simulink model "Zhongxiang_control"  (R2016a)
settings: Solver=VariableStepAuto  StartTime=0.0  StopTime=60  RelTol=1e-3
undefined symbols (not defined in the file or in its folder): aubr, tablebr, vubr
libraries: simulink x2, Solver_SF x1
settings Model: Creator=我  LastModifiedBy=我

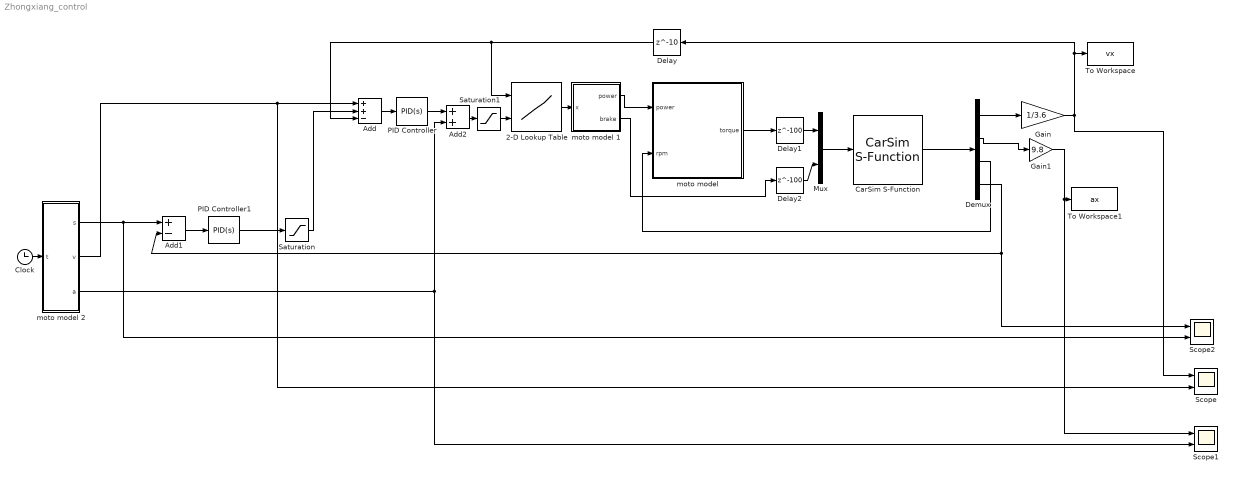
== system Zhongxiang_control ==
  2-D Lookup Table : Lookup_n-D  BreakpointsForDimension1=vubr  BreakpointsForDimension2=aubr  Table=tablebr  InternalRulePriority=Speed  RndMeth=Simplest  InputSameDT=on
  Add : Sum  Inputs=++-
  Add1 : Sum  Inputs=+-
  Add2 : Sum
  CarSim S-Function : Solver_SF/CarSim S-Function  Priority=1  SIMFILE=simfile.sim
  Clock : Clock
  Delay : Delay  DelayLength=10  InitialCondition=0
  Delay1 : Delay  DelayLength=100  InitialCondition=0  SampleTime=0.0001
  Delay2 : Delay  DelayLength=100  InitialCondition=0  SampleTime=0.0001
  Demux : Demux
  Gain : Gain  Gain=1/3.6
  Gain1 : Gain  Gain=9.8
  Mux : Mux  Inputs=2
  PID Controller : simulink/Continuous/PID Controller  Controller=PID  TimeDomain=Continuous-time  SampleTime=-1  IntegratorMethod=Forward Euler  FilterMethod=Forward Euler  Form=Parallel  UseFilter=on  ControllerParametersSource=internal  P=2  I=0.1  D=0.3  N=100  InitialConditionSource=internal  InitialConditionForIntegrator=0  InitialConditionForFilter=0  ExternalReset=none  LimitOutput=off  UpperSaturationLimit=inf  LowerSaturationLimit=-inf  LinearizeAsGain=on  AntiWindupMode=none  Kb=1  TrackingMode=off  Kt=1  PParamMin=[]  PParamMax=[]  IParamMin=[]  IParamMax=[]  DParamMin=[]  DParamMax=[]  NParamMin=[]  NParamMax=[]  KbParamMin=[]  KbParamMax=[]  KtParamMin=[]  KtParamMax=[]  POutMin=[]  POutMax=[]  IOutMin=[]  IOutMax=[]  DOutMin=[]  DOutMax=[]  NOutMin=[]  NOutMax=[]  KbOutMin=[]  KbOutMax=[]  KtOutMin=[]  KtOutMax=[]  IntegratorOutMin=[]  IntegratorOutMax=[]  FilterOutMin=[]  FilterOutMax=[]  SumOutMin=[]  SumOutMax=[]  SumI1OutMin=[]  SumI1OutMax=[]  SumI2OutMin=[]  SumI2OutMax=[]  SumI3OutMin=[]  SumI3OutMax=[]  SumDOutMin=[]  SumDOutMax=[]  SaturationOutMin=[]  SaturationOutMax=[]  IntegratorContinuousStateAttributes=''  IntegratorStateMustResolveToSignalObject=off  IntegratorRTWStateStorageClass=Auto  FilterContinuousStateAttributes=''  FilterStateMustResolveToSignalObject=off  FilterRTWStateStorageClass=Auto  DifferentiatorICPrevScaledInput=0  DifferentiatorOutMin=[]  DifferentiatorOutMax=[]
  PID Controller1 : simulink/Continuous/PID Controller  Controller=PID  TimeDomain=Continuous-time  SampleTime=-1  IntegratorMethod=Forward Euler  FilterMethod=Forward Euler  Form=Parallel  UseFilter=on  ControllerParametersSource=internal  P=2  I=0.1  D=0.3  N=100  InitialConditionSource=internal  InitialConditionForIntegrator=0  InitialConditionForFilter=0  ExternalReset=none  LimitOutput=off  UpperSaturationLimit=inf  LowerSaturationLimit=-inf  LinearizeAsGain=on  AntiWindupMode=none  Kb=1  TrackingMode=off  Kt=1  PParamMin=[]  PParamMax=[]  IParamMin=[]  IParamMax=[]  DParamMin=[]  DParamMax=[]  NParamMin=[]  NParamMax=[]  KbParamMin=[]  KbParamMax=[]  KtParamMin=[]  KtParamMax=[]  POutMin=[]  POutMax=[]  IOutMin=[]  IOutMax=[]  DOutMin=[]  DOutMax=[]  NOutMin=[]  NOutMax=[]  KbOutMin=[]  KbOutMax=[]  KtOutMin=[]  KtOutMax=[]  IntegratorOutMin=[]  IntegratorOutMax=[]  FilterOutMin=[]  FilterOutMax=[]  SumOutMin=[]  SumOutMax=[]  SumI1OutMin=[]  SumI1OutMax=[]  SumI2OutMin=[]  SumI2OutMax=[]  SumI3OutMin=[]  SumI3OutMax=[]  SumDOutMin=[]  SumDOutMax=[]  SaturationOutMin=[]  SaturationOutMax=[]  IntegratorContinuousStateAttributes=''  IntegratorStateMustResolveToSignalObject=off  IntegratorRTWStateStorageClass=Auto  FilterContinuousStateAttributes=''  FilterStateMustResolveToSignalObject=off  FilterRTWStateStorageClass=Auto  DifferentiatorICPrevScaledInput=0  DifferentiatorOutMin=[]  DifferentiatorOutMax=[]
  Saturation : Saturate  UpperLimit=10  LowerLimit=-10
  Saturation1 : Saturate  UpperLimit=5  LowerLimit=-8
  Scope : Scope  NumInputPorts=2
  Scope1 : Scope  NumInputPorts=2
  Scope2 : Scope  NumInputPorts=2
  To Workspace : ToWorkspace  VariableName=vx  SaveFormat=Timeseries  SampleTime=-1
  To Workspace1 : ToWorkspace  VariableName=ax  SaveFormat=Timeseries  SampleTime=-1
  "moto model " : MATLAB Function  TreatAsAtomicUnit=on
  moto model 1 : MATLAB Function  TreatAsAtomicUnit=on
  moto model 2 : MATLAB Function  TreatAsAtomicUnit=on
  wires:
  CarSim S-Function/1 -> Demux/1
  Gain1/1 -> To Workspace1/1, Scope1/1
  Mux/1 -> CarSim S-Function/1
  Gain/1 -> To Workspace/1, Delay/1, Scope/1
  Demux/1 -> Gain/1
  Demux/2 -> Gain1/1
  Demux/3 -> "moto model "/2(rpm)
  2-D Lookup Table/1 -> moto model 1/1(x)
  moto model 1/1(power) -> "moto model "/1(power)
  Add/1 -> PID Controller/1
  moto model 2/1(s) -> Scope2/2, Add1/1
  moto model 2/3(a) -> Add2/2, Scope1/2
  Add1/1 -> PID Controller1/1
  Demux/4 -> Scope2/1, Add1/2
  Clock/1 -> moto model 2/1(t)
  Delay/1 -> 2-D Lookup Table/1, Add/3
  PID Controller1/1 -> Saturation/1
  Saturation/1 -> Add/2
  PID Controller/1 -> Add2/1
  Add2/1 -> Saturation1/1
  Saturation1/1 -> 2-D Lookup Table/2
  moto model 2/2(v) -> Scope/2, Add/1
  "moto model "/1(torque) -> Delay1/1
  Delay1/1 -> Mux/1
  moto model 1/2(brake) -> Delay2/1
  Delay2/1 -> Mux/2

== matlab function Zhongxiang_control/moto model 1 ==
  data: x input; power output; brake output
function [power,brake]=fcn(x)
if (x>0)
    power=x;
    brake=0;
else
    brake=-x;
    power=0;
end

== matlab function Zhongxiang_control/moto model  ==
  data: power input; torque output; rpm input
function torque=fcn(power,rpm)
Tmax=380*power;
if (rpm<=4523)
    torque=Tmax;
else
    torque=(Tmax*4523)/rpm;
end
end

== matlab function Zhongxiang_control/moto model 2 ==
  data: t input; s output; v output; a output
function [s,v,a]=fcn(t)
 if t<10
     s=0.1*t^3/3;
     v=0.1*t^2;
     a=0.2*t;
 else
     a=2-0.1*(t-10);
     v=2*t-0.05*(t-10)^2-10;
     s=t^2-0.05*(t-10)^3/3-10*t+100/3;
 end
